simulink model "lotkavolterra2"  (R2014b)
settings: Solver=ode45  StartTime=0.0  StopTime=1000  RelTol=1e-3
settings Model: Creator=sigurd  LastModifiedBy=sigurd

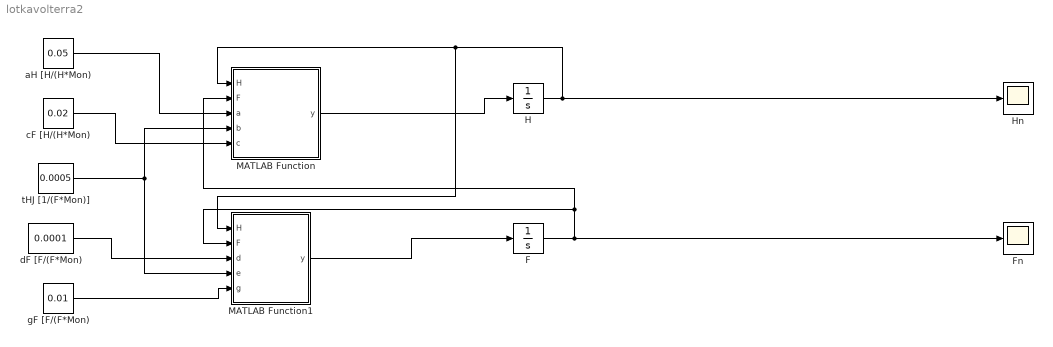
== system lotkavolterra2 ==
  F : Integrator  InitialCondition=50
  Fn : Scope
  H : Integrator  InitialCondition=200
  Hn : Scope
  MATLAB Function : MATLAB Function  TreatAsAtomicUnit=on
  MATLAB Function1 : MATLAB Function  TreatAsAtomicUnit=on
  aH [H/(H*Mon) : Constant  Value=0.05
  cF [H/(H*Mon) : Constant  Value=0.02
  dF [F/(F*Mon) : Constant  Value=0.0001
  gF [F/(F*Mon) : Constant  Value=0.01
  tHJ [1/(F*Mon)] : Constant  Value=0.0005
  wires:
  H/1 -> MATLAB Function1/1(H), MATLAB Function/1(H), Hn/1
  F/1 -> MATLAB Function1/2(F), MATLAB Function/2(F), Fn/1
  tHJ [1/(F*Mon)]/1 -> MATLAB Function/4(b), MATLAB Function1/4(e)
  gF [F/(F*Mon)/1 -> MATLAB Function1/5(g)
  dF [F/(F*Mon)/1 -> MATLAB Function1/3(d)
  cF [H/(H*Mon)/1 -> MATLAB Function/5(c)
  aH [H/(H*Mon)/1 -> MATLAB Function/3(a)
  MATLAB Function/1(y) -> H/1
  MATLAB Function1/1(y) -> F/1

== matlab function lotkavolterra2/MATLAB Function1 ==
  data: H input; y output; F input; d input; e input; g input
function y = fcn(H,F,d,e,g)
y = -(d*F)+(e*H*F)-(g*F*F);

== matlab function lotkavolterra2/MATLAB Function ==
  data: H input; y output; F input; a input; b input; c input
function y = fcn(H,F,a,b,c)
y = (a*H)-(b*H*F)-(c*H*H);
